simulink model "ps6"  (R2020b)
settings: Solver=VariableStepAuto  StartTime=0.0  StopTime=10.0  RelTol=1e-3
settings Model: Creator=prana  LastModifiedBy=prana

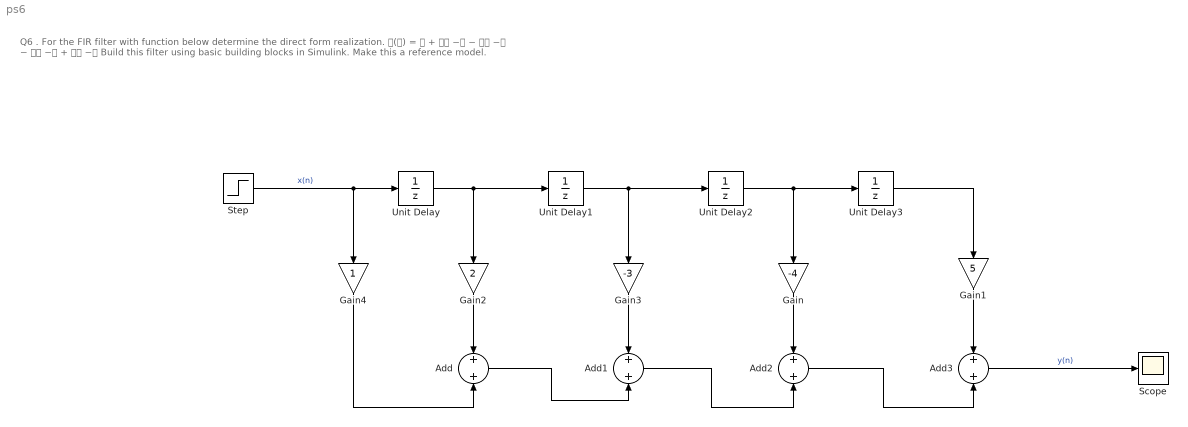
== system ps6 ==
  note: Q6 . For the FIR filter with function below determine the direct form realization. 𝐇(𝐳) = 𝟏 + 𝟐𝐳 −𝟏 − 𝟑𝐳 −𝟐 − 𝟒𝐳 −𝟑 + 𝟓𝐳 −𝟒 Build this filter using basic building blocks in Simulink. Make this a reference model.
  Add{,1..3} (4 alike) : Sum
  Gain : Gain  Gain=-4
  Gain1 : Gain  Gain=5
  Gain2 : Gain  Gain=2
  Gain3 : Gain  Gain=-3
  Gain4 : Gain
  Scope : Scope
  Step : Step  SampleTime=0
  Unit Delay{,1..3} (4 alike) : UnitDelay  SampleTime=-1  HasFrameUpgradeWarning=on
  wires:
  Unit Delay/1 -> Gain2/1, Unit Delay1/1
  Unit Delay1/1 -> Unit Delay2/1, Gain3/1
  Unit Delay2/1 -> Gain/1, Unit Delay3/1
  Step/1 -> Gain4/1, Unit Delay/1  "x(n)"
  Add/1 -> Add1/2
  Add1/1 -> Add2/2
  Add2/1 -> Add3/2
  Unit Delay3/1 -> Gain1/1
  Add3/1 -> Scope/1  "y(n)"
  Gain2/1 -> Add/1
  Gain3/1 -> Add1/1
  Gain/1 -> Add2/1
  Gain1/1 -> Add3/1
  Gain4/1 -> Add/2
